simulink model "motion_robot_dc_fal"  (Simulink 10.1)
settings: Solver=FixedStepAuto  StartTime=0.0  StopTime=60  FixedStep=fixedStep  MaxStep=0.2  RelTol=1e-3
values from neighbouring files (symbols this model uses):
  fixedStep = 1    [temperatureHumidityParametersInit.m]
  initT = 60    [temperatureHumidityParametersInit.m]
  maxT = 82    [heater2Init.m]
  minT = 70    [heater2Init.m]
undefined symbols (not defined in the file or in its folder): robotDis, sensitivityDis, Tdelta
settings Model: Creator=lixuansong  LastModifiedBy=ozgurozmen
settings DataIOCC: SaveOutput=off  SignalLogging=off  DSMLogging=off  SaveTime=off
settings OptimizationCC: LifeSpan=auto
settings DebuggingCC: UnderspecifiedInitializationDetection=Simplified  MergeDetectMultiDrivingBlocksExec=error  SFUnexpectedBacktrackingDiag=error  SFNoUnconditionalDefaultTransitionDiag=error  SFExecutionAtInitializationDiag=warning  ArithmeticOperatorsInVariantConditions=error
settings HardwareCC: ProdBitPerPointer=64  ProdBitPerSizeT=64  ProdBitPerPtrDiffT=64  ProdLargestAtomicFloat=Float  ProdIntDivRoundTo=Zero  ProdEndianess=LittleEndian  ProdWordSize=64  ProdHWDeviceType=Intel->x86-64 (Windows64)
settings ModelReferenceCC: PropagateSignalLabelsOutOfModel=on
settings SFSimCC: SimUseLocalCustomCode=on  CustomCodeUndefinedFunction=FilterOut
settings RTWCC: RTWUseLocalCustomCode=on
settings CodeAppCC: StateflowObjectComments=off
settings GRTTargetCC: TargetLangStandard=C99 (ISO)  CombineOutputUpdateFcns=on  GRTInterface=off
settings ConfigComp: CovMetricSettings=dwe  CovHtmlReporting=off  CovSaveCumulativeToWorkspaceVar=off  CovSaveSingleToWorkspaceVar=off  CovExternalEMLEnable=on

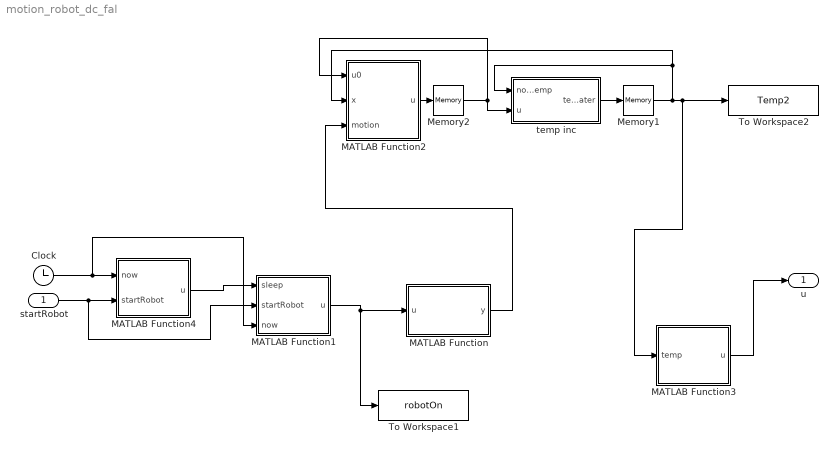
== system motion_robot_dc_fal ==
  startRobot : Inport
  Clock : Clock
  MATLAB Function : MATLAB Function  TreatAsAtomicUnit=on
  MATLAB Function1 : MATLAB Function  TreatAsAtomicUnit=on
  MATLAB Function2 : MATLAB Function  TreatAsAtomicUnit=on
  MATLAB Function3 : MATLAB Function  TreatAsAtomicUnit=on
  MATLAB Function4 : MATLAB Function  TreatAsAtomicUnit=on
  Memory1 : Memory  InitialCondition=initT
  Memory2 : Memory
  To Workspace1 : ToWorkspace  VariableName=robotOn  SampleTime=-1
  To Workspace2 : ToWorkspace  VariableName=Temp2  SampleTime=-1
  temp inc : MATLAB Function  TreatAsAtomicUnit=on
  u : Outport
  wires:
  Clock/1 -> MATLAB Function1/3(now), MATLAB Function4/1(now)
  startRobot/1 -> MATLAB Function1/2(startRobot), MATLAB Function4/2(startRobot)
  MATLAB Function4/1(u) -> MATLAB Function1/1(sleep)
  MATLAB Function1/1(u) -> MATLAB Function/1(u), To Workspace1/1
  MATLAB Function2/1(u) -> Memory2/1
  temp inc/1(tempHeater) -> Memory1/1
  Memory2/1 -> temp inc/2(u), MATLAB Function2/1(u0)
  MATLAB Function/1(y) -> MATLAB Function2/3(motion)
  Memory1/1 -> MATLAB Function2/2(x), temp inc/1(nowTemp), MATLAB Function3/1(temp), To Workspace2/1
  MATLAB Function3/1(u) -> u/1

== matlab function MATLAB Function1 ==
  data: u output double; sleep input double; timeSleep parameter double; startRobot input double; now input double
function u = controlRobot(sleep, timeSleep, startRobot, now)
if sleep == 1 && now<=startRobot+timeSleep
    u=1;
else
    u=0;
end

== matlab function MATLAB Function ==
  data: u input double; y output double; robotDis parameter double; sensitivityDis parameter double
function y = motionDetector(u, robotDis, sensitivityDis)

if robotDis<=sensitivityDis
    y=u;
else
    y=0;
end

== matlab function MATLAB Function2 ==
  data: u0 input double; x input double; u output double; minT parameter double; maxT parameter double; motion input double
function u = controlHeater(u0,x, minT, maxT,motion)


if motion == 1 && x < maxT
    u=1;
elseif x<minT 
    u=1;
elseif x>maxT
    u=0;
else 
    u=u0;
end

== matlab function temp inc ==
  data: tempHeater output double; Tdelta parameter double; nowTemp input double; u input double; fixedStep parameter double
function tempHeater = calcTemp(Tdelta, nowTemp, u,fixedStep)

td=Tdelta*fixedStep;

tempHeater=nowTemp+u*td;


end

== matlab function MATLAB Function4 ==
  data: u output double; now input double; timeSleep parameter double; startRobot input double
function u = controlMode(now,timeSleep, startRobot)
if now>=startRobot && now<=startRobot+timeSleep
    u=1;
else
    u=0;
end

== matlab function MATLAB Function3 ==
  data: u output double; temp input double
function u = controlLight(temp)
if temp>78
    u=1;
else
    u=0;
end
